simulink model "EPS_Simulation"  (R2018b)
settings: Solver=FixedStepAuto  StartTime=0.0  StopTime=10.0  FixedStep=0.01  RelTol=1e-3
undefined symbols (not defined in the file or in its folder): sigbuilder_block
settings Model: PauseTimes=2  Creator=ADMIN  LastModifiedBy=ADMIN
settings SolverCC: AlgebraicLoopSolver=LineSearch

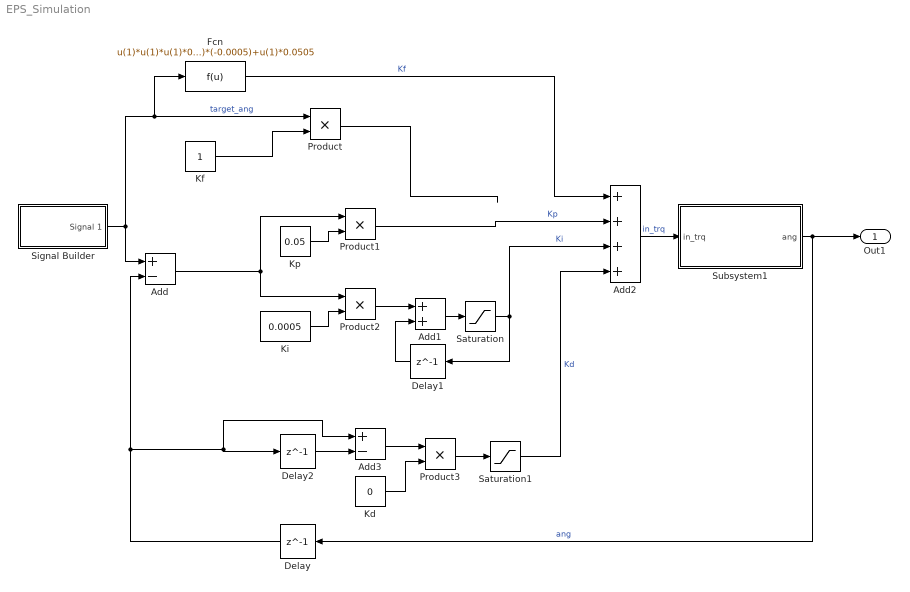
== system EPS_Simulation ==
  Add : Sum  Inputs=+-
  Add1 : Sum
  Add2 : Sum  Inputs=++++
  Add3 : Sum  Inputs=+-
  Delay : Delay  DelayLength=1
  Delay1 : Delay  DelayLength=1
  Delay2 : Delay  DelayLength=1
  Fcn : Fcn  Expr=u(1)*u(1)*u(1)*0.000002+u(1)*u(1)*(-0.0005)+u(1)*0.0505
  Kd : Constant  Value=0
  Kf : Constant
  Ki : Constant  Value=0.0005
  Kp : Constant  Value=0.05
  Product{,1..3} (4 alike) : Product
  Saturation : Saturate
  Saturation1 : Saturate  UpperLimit=1  LowerLimit=-0.1
  Signal Builder : Subsystem  Tag=STV Subsys  LoadFcn=sigbuilder_block('load');  StartFcn=sigbuilder_block('start');  StopFcn=sigbuilder_block('stop');  ClipboardFcn=sigbuilder_block('clipboard');  mask(Sigbuilder block){tuvar=[0:10]}
      mask help: Simulink:masks:SigbuilderBlock_MD
      mask init:
      | if ~strcmp(get_param(bdroot(gcbh),'SimulationStatus'),'stopped') tuvar = sigbuilder_block('maskInit'); end
      settings: CopyFcn=sigbuilder_block('copy');  DeleteFcn=sigbuilder_block('delete');  ModelCloseFcn=sigbuilder_block('modelClose');  PreSaveFcn=sigbuilder_block('preSave');  PauseFcn=sigbuilder_block('pause');  ContinueFcn=sigbuilder_block('continue');  NameChangeFcn=sigbuilder_block('namechange');  OpenFcn=sigbuilder_block('open',[437.6 199.2 550.4 400 ]);  CloseFcn=sigbuilder_block('close');
      mask Display: plot(0, 0, 100, 100,[2, 2, 32, 32, 2], [68, 8, 8, 68, 68],[32, 2], [38, 38], [32, 19, 2],[53, 60, 44], [32, 17, 17, 2],[16, 16, 31, 31]);txt = getActiveGroup(gcbh);text(2, 100, txt,'verticalAlignment', 'top');
  Subsystem1 : Subsystem
  Out1 : Outport
  wires:
  Product1/1 -> Add2/2  "Kp"
  Subsystem1/1(ang) -> Delay/1, Out1/1  "ang"
  Signal Builder/1(Signal 1) -> Fcn/1, Product/1, Add/1  "target_ang"
  Kf/1 -> Product/2
  Add/1 -> Product2/1, Product1/1
  Kp/1 -> Product1/2
  Ki/1 -> Product2/2
  Product2/1 -> Add1/1
  Add1/1 -> Saturation/1
  Delay1/1 -> Add1/2
  Saturation/1 -> Delay1/1, Add2/3  "Ki"
  Product/1 -> ?
  Add2/1 -> Subsystem1/1(in_trq)  "in_trq"
  Delay2/1 -> Add3/2
  Add3/1 -> Product3/1
  Kd/1 -> Product3/2
  Product3/1 -> Saturation1/1
  Fcn/1 -> Add2/1  "Kf"
  Saturation1/1 -> Add2/4  "Kd"
  Delay/1 -> Delay2/1, Add3/1, Add/2

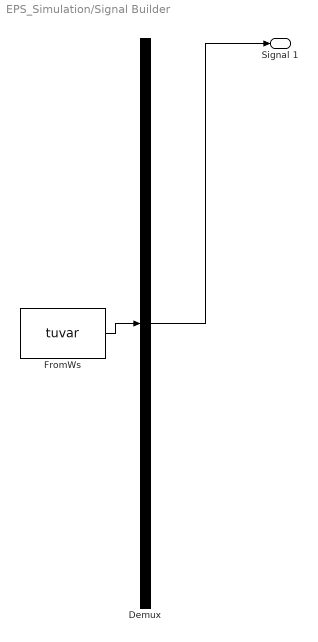
== system EPS_Simulation/Signal Builder ==
  Demux : Demux  Tag=STV Demux  Outputs=1
  FromWs : FromWorkspace  Tag=STV FromWs  VariableName=tuvar  SampleTime=0
      SigBuilderData=|
      | common.afterFinalStr = 'Extrapolate'
      | common.sampleTime = 0
      | dataSet.timeRange = [0 10]
      | dataSet.name = 'Group 1'
      | sbobj.Groups.Name = 'Group 1'
      | sbobj.Groups.Signals.Name = 'Signal 1'
      | sbobj.Groups.Signals.XData = [0 2 2 3.56 8.44 10]
      | sbobj.Groups.Signals.YData = [0 0 29.4 3.8 -4.4 30]
  Signal 1 : Outport  Tag=STV Outport
  wires:
  Demux/1 -> Signal 1/1
  FromWs/1 -> Demux/1

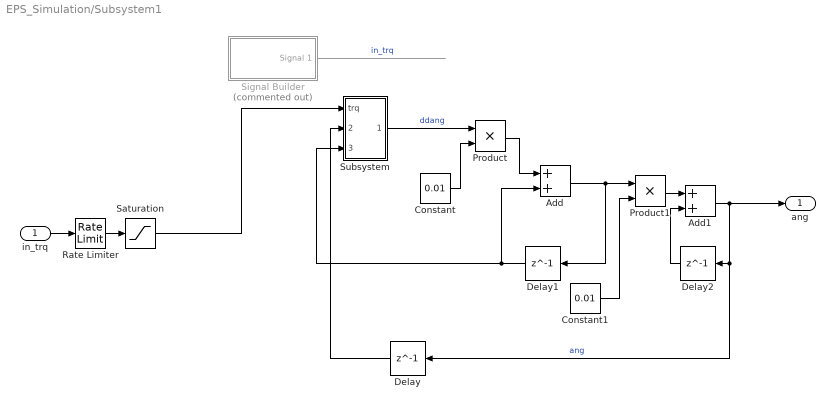
== system EPS_Simulation/Subsystem1 ==
  in_trq : Inport
  Add : Sum
  Add1 : Sum
  Constant : Constant  Value=0.01
  Constant1 : Constant  Value=0.01
  Delay : Delay  DelayLength=1
  Delay1 : Delay  DelayLength=1
  Delay2 : Delay  DelayLength=1
  Product : Product
  Product1 : Product
  Rate Limiter : RateLimiter  RisingSlewLimit=10  FallingSlewLimit=-10  SampleTimeMode=inherited
  Saturation : Saturate  UpperLimit=2  LowerLimit=-2
  Signal Builder : Subsystem  Tag=STV Subsys  Commented=on  LoadFcn=sigbuilder_block('load');  StartFcn=sigbuilder_block('start');  StopFcn=sigbuilder_block('stop');  ClipboardFcn=sigbuilder_block('clipboard');  mask(Sigbuilder block){tuvar=[0:10]}
      mask help: Simulink:masks:SigbuilderBlock_MD
      mask init:
      | if ~strcmp(get_param(bdroot(gcbh),'SimulationStatus'),'stopped') tuvar = sigbuilder_block('maskInit'); end
      settings: CopyFcn=sigbuilder_block('copy');  DeleteFcn=sigbuilder_block('delete');  ModelCloseFcn=sigbuilder_block('modelClose');  PreSaveFcn=sigbuilder_block('preSave');  PauseFcn=sigbuilder_block('pause');  ContinueFcn=sigbuilder_block('continue');  NameChangeFcn=sigbuilder_block('namechange');  OpenFcn=sigbuilder_block('open',[437.6 199.2 550.4 400 ]);  CloseFcn=sigbuilder_block('close');
      mask Display: plot(0, 0, 100, 100,[2, 2, 32, 32, 2], [68, 8, 8, 68, 68],[32, 2], [38, 38], [32, 19, 2],[53, 60, 44], [32, 17, 17, 2],[16, 16, 31, 31]);txt = getActiveGroup(gcbh);text(2, 100, txt,'verticalAlignment', 'top');
  Subsystem : Subsystem
  ang : Outport
  wires:
  Constant1/1 -> Product1/2
  Subsystem/1(Out1) -> Product/1  "ddang"
  Add1/1 -> ang/1, Delay2/1, Delay/1  "ang"
  Constant/1 -> Product/2
  Product/1 -> Add/1
  Delay2/1 -> Add1/2
  Delay/1 -> Subsystem/2(ang)
  Delay1/1 -> Add/2, Subsystem/3(angspd)
  Add/1 -> Delay1/1, Product1/1
  Product1/1 -> Add1/1
  in_trq/1 -> Rate Limiter/1
  Signal Builder/1(Signal 1) -> ?  "in_trq"
  Rate Limiter/1 -> Saturation/1
  Saturation/1 -> Subsystem/1(trq)

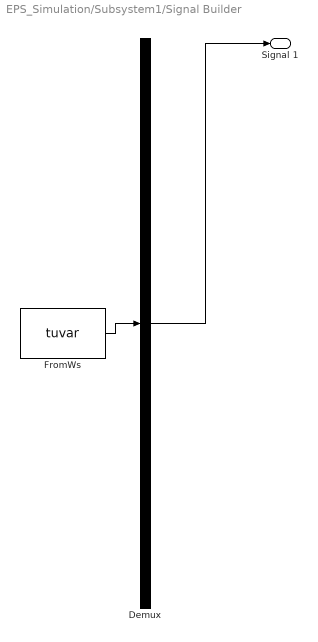
== system EPS_Simulation/Subsystem1/Signal Builder ==
  Demux : Demux  Tag=STV Demux  Outputs=1
  FromWs : FromWorkspace  Tag=STV FromWs  VariableName=tuvar  SampleTime=0
      SigBuilderData=|
      | common.afterFinalStr = 'Extrapolate'
      | common.sampleTime = 0
      | dataSet.timeRange = [0 10]
      | dataSet.name = 'Group 1'
      | sbobj.Groups.Name = 'Group 1'
      | sbobj.Groups.Signals.Name = 'Signal 1'
      | sbobj.Groups.Signals.XData = [0 2.24 5 6.02 10]
      | sbobj.Groups.Signals.YData = [0 -0.72 1.695 -1.56 0.5]
  Signal 1 : Outport  Tag=STV Outport
  wires:
  Demux/1 -> Signal 1/1
  FromWs/1 -> Demux/1

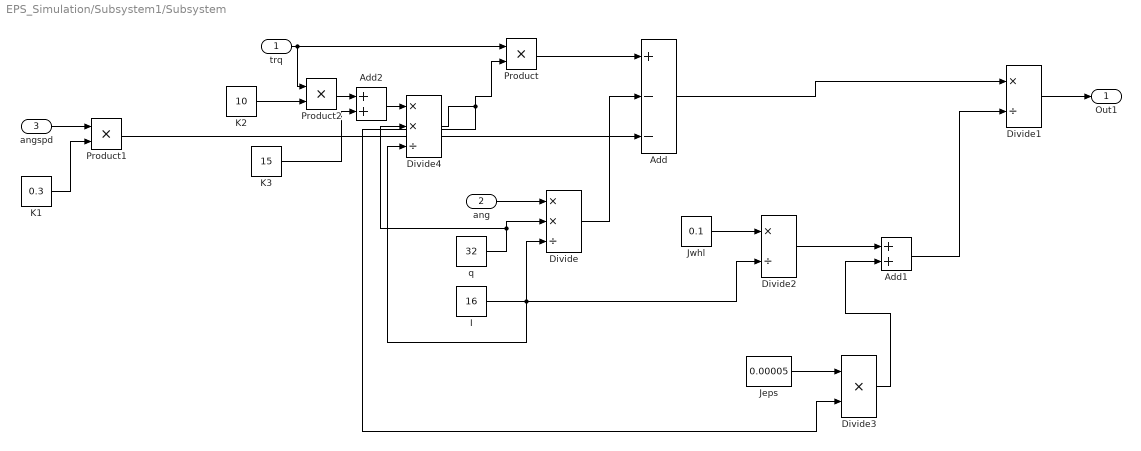
== system EPS_Simulation/Subsystem1/Subsystem ==
  trq : Inport
  ang : Inport  Port=2
  angspd : Inport  Port=3
  Add : Sum  Inputs=+--
  Add1 : Sum
  Add2 : Sum
  Divide : Product  Inputs=**/
  Divide1 : Product  Inputs=*/
  Divide2 : Product  Inputs=*/
  Divide3 : Product  Inputs=**
  Divide4 : Product  Inputs=**/
  I : Constant  Value=16
  Jeps : Constant  Value=0.00005
  Jwhl : Constant  Value=0.1
  K1 : Constant  Value=0.3
  K2 : Constant  Value=10
  K3 : Constant  Value=15
  Product : Product
  Product1 : Product
  Product2 : Product
  q : Constant  Value=32
  Out1 : Outport
  wires:
  trq/1 -> Product2/1, Product/1
  Product/1 -> Add/1
  Divide1/1 -> Out1/1
  Add/1 -> Divide1/1
  Add1/1 -> Divide1/2
  ang/1 -> Divide/1
  q/1 -> Divide/2, Divide4/2
  Divide/1 -> Add/2
  Jwhl/1 -> Divide2/1
  I/1 -> Divide/3, Divide4/3, Divide2/2
  Divide2/1 -> Add1/1
  Divide4/1 -> Product/2, Divide3/2
  Jeps/1 -> Divide3/1
  Divide3/1 -> Add1/2
  angspd/1 -> Product1/1
  Product1/1 -> Add/3
  K1/1 -> Product1/2
  K2/1 -> Product2/2
  Product2/1 -> Add2/1
  K3/1 -> Add2/2
  Add2/1 -> Divide4/1
